simulink model "sampleModel302"  (R2021b)
settings: Solver=VariableStepAuto  StartTime=0.0  StopTime=10.0  RelTol=1e-3
undefined symbols (not defined in the file or in its folder): Newton, Raphson
settings Model: Creator=user  LastModifiedBy=user

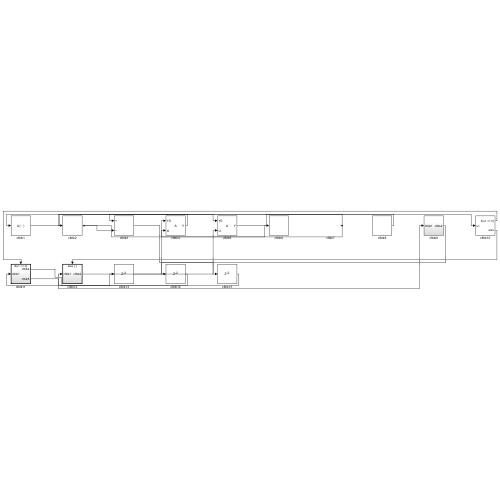
[thumbnail: Simulink's stored preview of the top-level diagram]
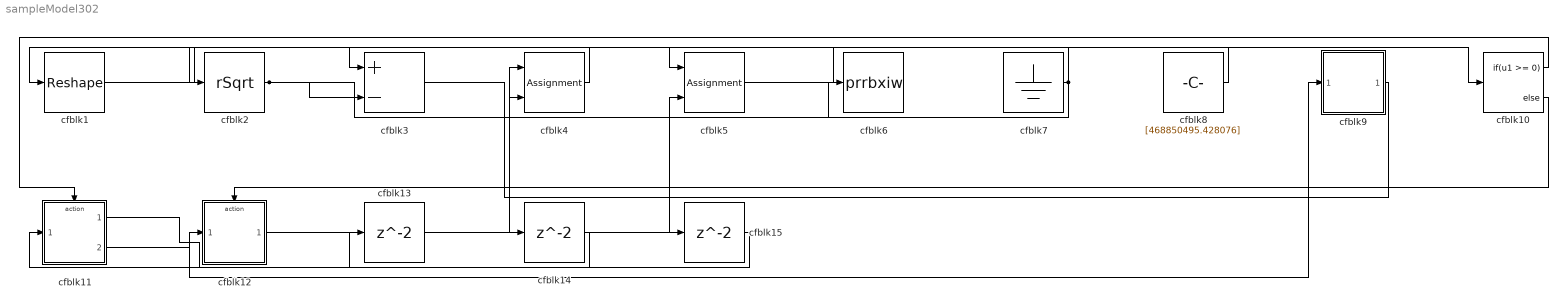
== system sampleModel302 ==
  cfblk1 : Reshape
  cfblk10 : If  IfExpression=u1 >= 0  SampleTime=1
  cfblk11 : Subsystem  TreatAsAtomicUnit=on
  cfblk12 : Subsystem  TreatAsAtomicUnit=on
  cfblk13 : Delay  SampleTime=1
  cfblk14 : Delay  SampleTime=1
  cfblk15 : Delay  SampleTime=1
  cfblk2 : Sqrt  Operator=rSqrt  AlgorithmType=Newton-Raphson  SaturateOnIntegerOverflow=on
  cfblk3 : Sum  Inputs=+-
  cfblk4 : Assignment  DiagnosticForDimensions=Warning  IndexOptions=Index vector (dialog)  Indices=1  OutputSizes=1
  cfblk5 : Assignment  DiagnosticForDimensions=Warning  IndexOptions=Index vector (dialog)  Indices=1  OutputSizes=1
  cfblk6 : ToWorkspace  VariableName=prrbxiw  SaveFormat=Timeseries  SampleTime=-1
  cfblk7 : Ground
  cfblk8 : Constant  Value=[468850495.428076]  SampleTime=1
  cfblk9 : Subsystem
  wires:
  cfblk12/1(cfblk2) -> cfblk4/1
  cfblk1/1 -> cfblk5/1
  cfblk5/1 -> cfblk10/1
  cfblk8/1 -> cfblk3/1
  cfblk7/1 -> cfblk4/2, cfblk1/1
  cfblk4/1 -> cfblk2/1
  cfblk11/2(cfblk5) -> cfblk9/1(cfblk1)
  cfblk2/1 -> cfblk6/1, cfblk3/2
  cfblk10/1 -> cfblk11/Action
  cfblk10/2 -> cfblk12/Action
  cfblk11/1(cfblk2) -> cfblk13/1
  cfblk13/1 -> cfblk5/2
  cfblk9/1(cfblk2) -> cfblk14/1
  cfblk14/1 -> cfblk11/1(cfblk1)
  cfblk3/1 -> cfblk15/1
  cfblk15/1 -> cfblk12/1(cfblk1)

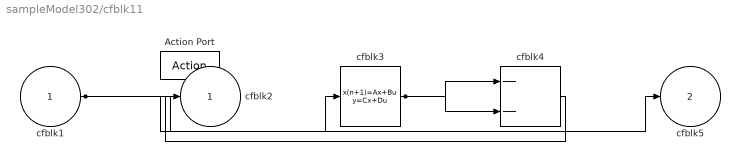
== system sampleModel302/cfblk11 ==
  cfblk1 : Inport
  Action Port : ActionPort  ActionPortLabel=if(u1 >= 0)
  cfblk3 : DiscreteStateSpace  SampleTime=-1
  cfblk4 : Sum  Inputs=--
  cfblk2 : Outport
  cfblk5 : Outport  Port=2
  wires:
  cfblk1/1 -> cfblk3/1, cfblk5/1
  cfblk3/1 -> cfblk4/1, cfblk4/2
  cfblk4/1 -> cfblk2/1

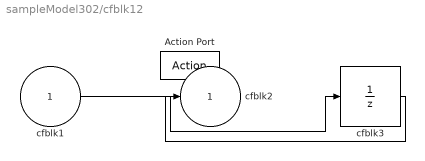
== system sampleModel302/cfblk12 ==
  cfblk1 : Inport
  Action Port : ActionPort  ActionPortLabel=else
  cfblk3 : UnitDelay  SampleTime=-1  HasFrameUpgradeWarning=on
  cfblk2 : Outport
  wires:
  cfblk1/1 -> cfblk3/1
  cfblk3/1 -> cfblk2/1

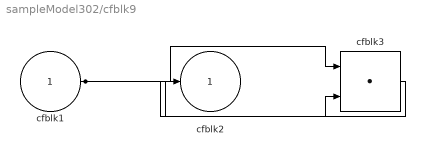
== system sampleModel302/cfblk9 ==
  cfblk1 : Inport
  cfblk3 : DotProduct  InputSameDT=on  OutDataTypeStr=Inherit: Inherit via internal rule
  cfblk2 : Outport
  wires:
  cfblk1/1 -> cfblk3/1, cfblk3/2
  cfblk3/1 -> cfblk2/1
